simulink model "auto_dataType_Error"  (R2017b)
settings: Solver=FixedStepDiscrete  StartTime=0.0  StopTime=10.0  FixedStep=0.200000  RelTol=1e-3  EnableMultiTasking=on
PreLoadFcn:
  | cellInfo =  {  { ...
  |    'ECI_state_msg', ...
  |    '', ...
  | sprintf(''), { ...
  |    {'r_ECI', 3, 'double', -1, 'real', 'Sample'}; ...
  |  {'v_ECI', 3, 'double', -1, 'real', 'Sample'}; ...
  |    }  } };
  | Simulink.Bus.cellToObject(cellInfo);
settings Model: Creator=hbourbou  LastModifiedBy=hbourbou
settings DataIOCC: LimitDataPoints=on  SaveFormat=Structure
settings OptimizationCC: LifeSpan=inf
settings DebuggingCC: SFUnexpectedBacktrackingDiag=warning  SFNoUnconditionalDefaultTransitionDiag=warning  SFExecutionAtInitializationDiag=none
settings HardwareCC: ProdBitPerPointer=32  ProdBitPerSizeT=32  ProdBitPerPtrDiffT=32  ProdLargestAtomicFloat=None  ProdIntDivRoundTo=Undefined  ProdEndianess=Unspecified  ProdWordSize=32  ProdHWDeviceType=32-bit Generic
settings ModelReferenceCC: PropagateSignalLabelsOutOfModel=off
settings CodeAppCC: StateflowObjectComments=on
settings GRTTargetCC: TargetLangStandard=C89/C90 (ANSI)  GeneratePreprocessorConditionals=Disable all
settings ConfigComp: CovMetricSettings=dw  CovHtmlReporting=on  CovSaveCumulativeToWorkspaceVar=on  CovSaveSingleToWorkspaceVar=on  CovExternalEMLEnable=off

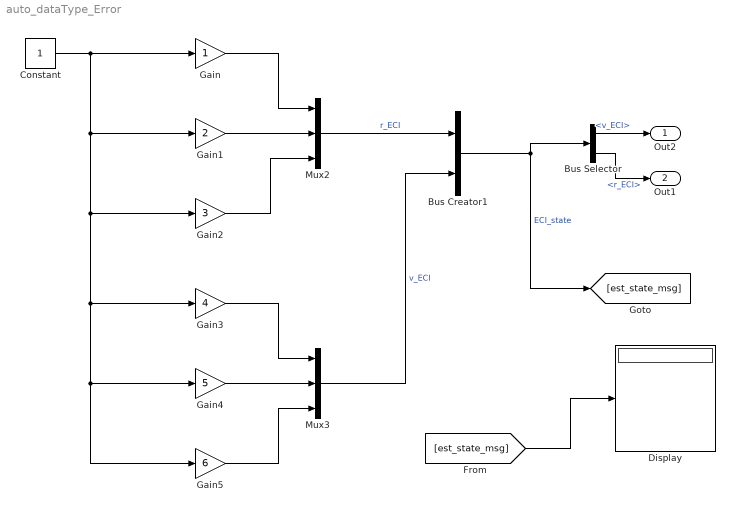
== system auto_dataType_Error ==
  Bus Creator1 : BusCreator  Inputs=2
  Bus Selector : BusSelector  OutputSignals=v_ECI,r_ECI
  Constant : Constant
  Display : Display
  Gain : Gain
  Gain1 : Gain  Gain=2
  Gain2 : Gain  Gain=3
  Gain3 : Gain  Gain=4
  Gain4 : Gain  Gain=5
  Gain5 : Gain  Gain=6
  Mux2 : Mux  Inputs=3
  Mux3 : Mux  Inputs=3
  Out2 : Outport
  Out1 : Outport  Port=2
  wires:
  Mux3/1 -> Bus Creator1/2  "v_ECI"
  Constant/1 -> Gain/1, Gain1/1, Gain2/1, Gain3/1, Gain5/1, Gain4/1
  Gain1/1 -> Mux2/2
  Mux2/1 -> Bus Creator1/1  "r_ECI"
  Bus Creator1/1 -> Bus Selector/1, [est_state_msg]  "ECI_state"
  Gain2/1 -> Mux2/3
  Gain/1 -> Mux2/1
  [est_state_msg] -> Display/1
  Bus Selector/2 -> Out1/1  "<r_ECI>"
  Bus Selector/1 -> Out2/1  "<v_ECI>"
  Gain3/1 -> Mux3/1
  Gain4/1 -> Mux3/2
  Gain5/1 -> Mux3/3
